simulink model "phase_ref"  (R2015b)
settings: Solver=VariableStepAuto  StartTime=0.0  StopTime=10.0  RelTol=1e-3
libraries: powerlib x3, powerlib_meascontrol x1
settings Model: Creator=kad  LastModifiedBy=kad

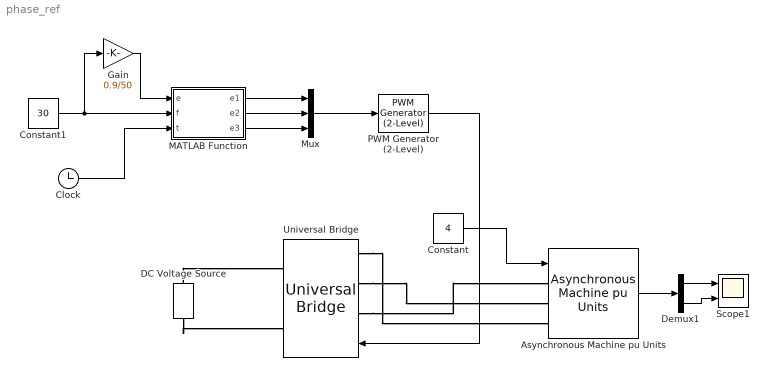
== system phase_ref ==
  Asynchronous Machine pu Units : powerlib/Machines/Asynchronous Machine pu Units  RotorType=Squirrel-cage  PresetModel=No  MechanicalLoad=Torque Tm  ShowDetailedParameters=on  ReferenceFrame=Rotor  Units=pu  MeasurementBus=off  NominalParameters=[3730 460 60]  Stator=[0.01965 0.0397]  Rotor=[0.01909 0.0397]  Cage1=[0.01909 0.0397]  Cage2=[0.01909 0.0397]  Lm=1.354  Mechanical=[0.09526 0.05479 2]  PolePairs=2  InitialConditions="[ 1,0   0,0,0   0,0,0 ]"  SimulateSaturation=off  Saturation="[0.212,0.4201,0.8125,1.0979,1.4799,2.2457,3.2586,4.5763,6.4763 ;   0.5,0.7,0.9,1,1.1,1.2 ,1.3,1.4,1.5]"  LoadFlowParameters=0  TsPowergui=0  TsBlock=-1  IterativeModel=Trapezoidal non iterative  Pmec=0
  Clock : Clock
  Constant : Constant  Value=4
  Constant1 : Constant  Value=30
  DC Voltage Source : powerlib/Electrical Sources/DC Voltage Source  Amplitude=100  Measurements=None
  Demux1 : Demux  Outputs=2
  Gain : Gain  Gain=0.9/50
  MATLAB Function : MATLAB Function  TreatAsAtomicUnit=on
  Mux : Mux  Inputs=3
  PWM Generator (2-Level) : powerlib_meascontrol/Pulse & Signal Generators/PWM Generator (2-Level)  ModulatorType=Three-phase bridge (6 pulses)  ModulatorMode=Unsynchronized  Fc=1000  Pc=90  nF=27  MinMax="[ -1  1 ]"  SamplingTechnique=Symmetrical regular (single edge)  ModulatingSignals=off  m=0.8  Freq=60  Phase=0  Ts=1e6  ShowCarrierOutport=off
  Scope1 : Scope  NumInputPorts=2
  Universal Bridge : powerlib/Power Electronics/Universal Bridge  Arms=3  SnubberResistance=1e5  SnubberCapacitance=inf  Device=IGBT / Diodes  Ron=1e-3  Lon=0  ForwardVoltages="[  0  0  ]"  ForwardVoltage=0  GTOparameters=[ 10e-6 , 20e-6 ]  IGBTparameters=[ 1e-6 , 2e-6 ]  Measurements=None  Measurements_2=None  converterType=Rectifier
  wires:
  Constant/1 -> Asynchronous Machine pu Units/1
  MATLAB Function/1(e1) -> Mux/1
  MATLAB Function/2(e2) -> Mux/2
  MATLAB Function/3(e3) -> Mux/3
  Mux/1 -> PWM Generator (2-Level)/1
  Clock/1 -> MATLAB Function/3(t)
  Constant1/1 -> Gain/1, MATLAB Function/2(f)
  PWM Generator (2-Level)/1 -> Universal Bridge/1
  Gain/1 -> MATLAB Function/1(e)
  Asynchronous Machine pu Units/1 -> Demux1/1
  Demux1/1 -> Scope1/1
  Demux1/2 -> Scope1/2
  connections:
  DC Voltage Source/RConn1 -- Universal Bridge/RConn1
  DC Voltage Source/LConn1 -- Universal Bridge/RConn2
  Universal Bridge/LConn1 -- Asynchronous Machine pu Units/LConn1
  Universal Bridge/LConn2 -- Asynchronous Machine pu Units/LConn2
  Universal Bridge/LConn3 -- Asynchronous Machine pu Units/LConn3

== matlab function phase_ref/MATLAB Function ==
  data: e input; e1 output; f input; t input; e2 output; e3 output
function [e1,e2,e3] = fcn(e,f,t)
%#codegen

e1=e*sin(2*pi*f*t);
e2=e*sin(2*pi*f*t-2*pi/3);
e3=e*sin(2*pi*f*t-4*pi/3);
